simulink model "Esquiva"  (R2023b)
settings: Solver=FixedStepAuto  StartTime=0.0  StopTime=inf  RelTol=1e-3  EnableMultiTasking=on
settings Model: ExtModeTrigDuration=2  Creator=Usuario_UMA  LastModifiedBy=alumnos
settings OptimizationCC: EnhancedBackFolding=on  PassReuseOutputArgsAs=Individual arguments  ZeroExternalMemoryAtStartup=off  ZeroInternalMemoryAtStartup=off  MaxStackSize=64  OptimizeBlockOrder=speed  DifferentSizesBufferReuse=on  OptimizationCustomize=off  EfficientTunableParamExpr=on
settings DebuggingCC: ParameterTunabilityLossMsg=error
settings HardwareCC: ProdBitPerInt=16  ProdBitPerPointer=16  ProdBitPerSizeT=16  ProdBitPerPtrDiffT=16  ProdLargestAtomicFloat=None  ProdWordSize=8  ProdHWDeviceType=Atmel->AVR
settings SFSimCC: MATLABDynamicMemAlloc=off
settings RTWCC: Description=Embedded Coder  SystemTargetFile=ert.tlc  HardwareBoard=Arduino Mega 2560  TemplateMakefile=ert_default_tmf  Toolchain=Arduino AVR  BuildConfiguration=Faster Runs
settings CodeAppCC: ForceParamTrailComments=on  IgnoreCustomStorageClasses=off  OperatorAnnotations=on  SimulinkDataObjDesc=on  SFDataObjDesc=on  InsertBlockDesc=on
settings ERTTargetCC: SupportContinuousTime=on  SupportVariableSizeSignals=on  ExtModeTransport=3  ExtModeStaticAlloc=on  ExtModeAutomaticAllocSize=off  ExtModeStaticAllocSize=2048  ExtModeMexFile=ext_xcp  ExtModeIntrfLevel=Level2 - Open

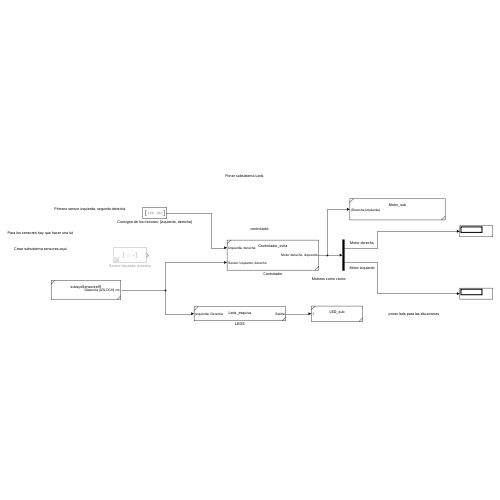
[thumbnail: Simulink's stored preview of the top-level diagram]
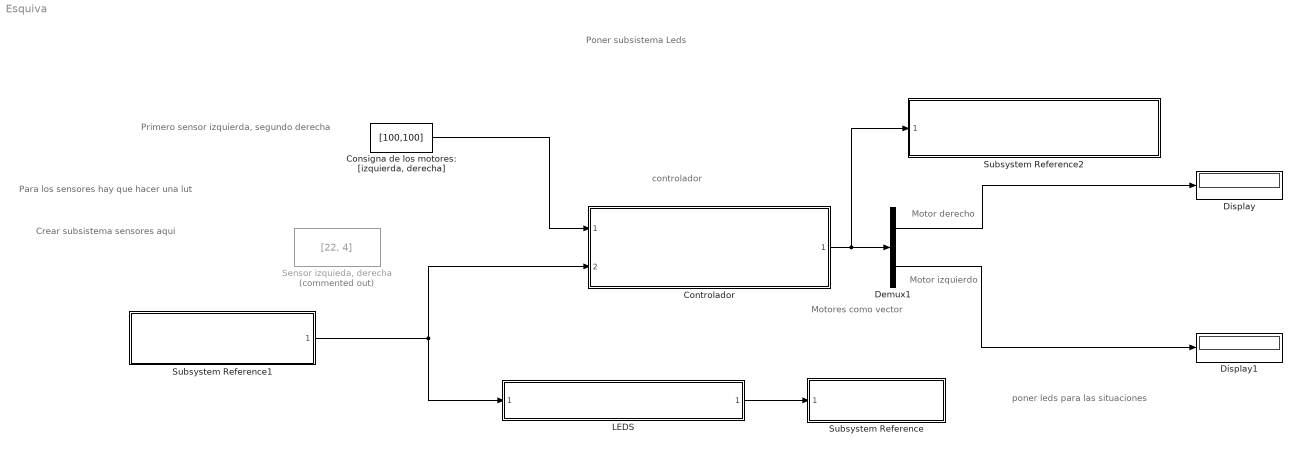
== system Esquiva ==
  note: Motor derecho
  note: Primero sensor izquierda, segundo derecha
  note: Para los sensores hay que hacer una lut
  note: poner leds para las situaciones
  note: Motores como vector
  note: controlador
  note: Poner subsistema Leds
  note: Crear subsistema sensores aqui
  note: Motor izquierdo
  "Consigna de los motores: [izquierda, derecha]" : Constant  Value=[100,100]
  Controlador : Subsystem  ReferencedSubsystem=Controlador_evita
  Demux1 : Demux  Outputs=2
  Display : Display
  Display1 : Display
  LEDS : Subsystem  ReferencedSubsystem=Leds_esquiva
  "Sensor izquieda, derecha" : Constant  Commented=on  Value=[22, 4]
  Subsystem Reference : Subsystem  ReferencedSubsystem=LED_sub
  Subsystem Reference1 : Subsystem  ReferencedSubsystem=subsysSensoresIR
  Subsystem Reference2 : Subsystem  ReferencedSubsystem=Motor_sub
  wires:
  "Consigna de los motores: [izquierda, derecha]"/1 -> Controlador/1
  Controlador/1 -> Subsystem Reference2/1, Demux1/1
  Demux1/2 -> Display1/1
  Demux1/1 -> Display/1
  LEDS/1 -> Subsystem Reference/1
  Subsystem Reference1/1 -> LEDS/1, Controlador/2
